simulink model "pam4"  (R2024a)
settings: Solver=VariableStepAuto  StartTime=0.0  StopTime=1  RelTol=1e-3
values from neighbouring files (symbols this model uses):
  channelCoeffs = [0.7,-0.2,0.1,0.3,0.2,-0.1]    [init.m]
  delay = span/2*M    (= 2)    [init.m]
  h = h/max(h)    [init.m]
  Rb = Rs*M    (= 7680000000)    [init.m]
  sps = 4    [init.m]
libraries: commdigbbndam3 x2, commchan3 x1, commrandsrc3 x1, commsink2 x1, dspadpt3 x1, dspsigops x1
settings Model: Creator=abc  LastModifiedBy=abc

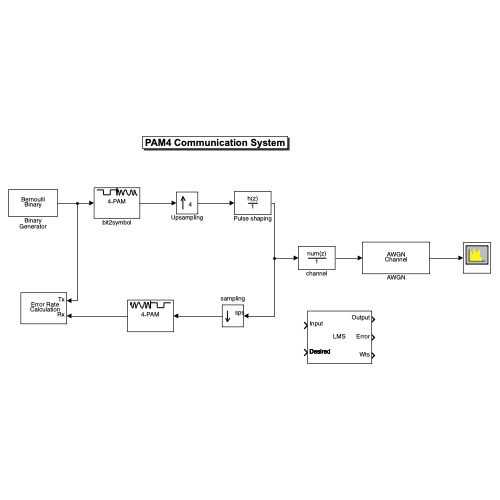
[thumbnail: Simulink's stored preview of the top-level diagram]
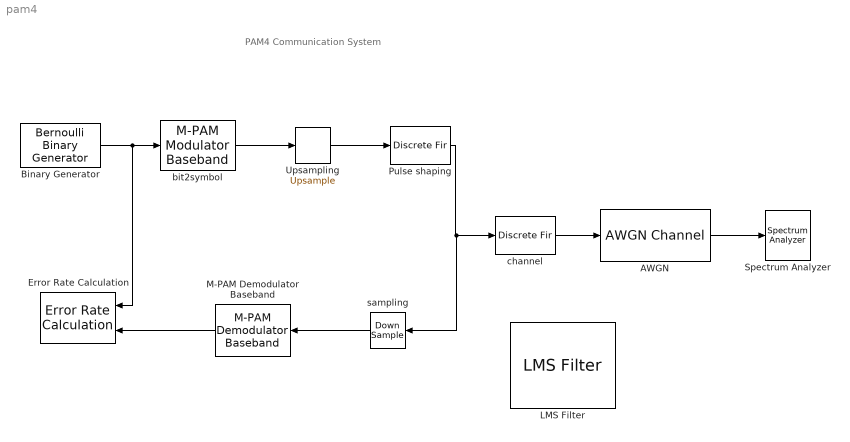
== system pam4 ==
  note: PAM4 Communication System
  AWGN : commchan3/AWGN Channel  LegacyMode=off  NoiseMethod="Signal to noise ratio  (Eb/No)"  noiseMode="Signal to noise ratio  (SNR)"  EbNo=EbN0  EsNo=10  SNR=10  BitsPerSymbol=M  SignalPower=signalPower  SamplesPerSymbol=sps  SymbolPeriod=1  VarianceSource=Parameter  Variance=1  RandomStream=Global stream  Seed=67  SimulateUsing=Interpreted execution
  Binary Generator : commrandsrc3/Bernoulli Binary Generator  ProbabilityOfZero=0.5  SeedSource=Auto  Seed=0  SampleTime=1/Rb  SamplesPerFrame=batchSize  OutputDataType=boolean  SimulateUsing=Interpreted execution
  Error Rate Calculation : commsink2/Error Rate Calculation  N=delay  st_delay=0  cp_mode=Entire frame  subframe=[]  PMode=Workspace  WsName=ErrorVec  RsMode2=off  stop=off  numErr=100  maxBits=1e6
  LMS Filter : dspadpt3/LMS Filter  Algo=LMS  L=16  stepflag=Dialog  mu=0.01  leakage=1.0  ic=0  Adapt=off  resetflag=None  weights=on  addnparflag=off  roundingMode=Floor  overflowMode=off
  M-PAM Demodulator Baseband : commdigbbndam3/M-PAM Demodulator Baseband  M=4  OutType=Bit  Dec=Gray  PowType=Min. distance between symbols  MinDist=2  AvgPow=1  PeakPow=1  outDtype1=boolean  outDtype2=Inherit via internal rule  denormFactorWordLen=16  denormFactorDataTypeStr=Inherit: Same word length as input  denormFactorLastDataTypeStr=Inherit: Same word length as input  prodOutWordLen=16  prodOutRoundingMode=Floor  prodOutOverflowMode=Wrap  prodOutOvFlMode=off  prodOutOvFlModeLastStrValue=off  sumWordLen=16
  Pulse shaping : DiscreteFir  Coefficients=h  InputProcessing=Columns as channels (frame based)
  Spectrum Analyzer : SpectrumAnalyzer  WindowPosition=[454.000000,177.000000,800.000000,500.000000,]  ScopeFrameLocation=window  Span=61440000000  StartFrequency=-30720000000  StopFrequency=30720000000  YLimits=[-73.48980676,24.64167876]
  Upsampling : dspsigops/Upsample  FactorSource=Dialog parameter  N=sps  Nmax=16  phase=0  InputProcessing=Columns as channels (frame based)  RateOptions=Enforce single-rate processing  ic=0  mode=Unused parameter value
  bit2symbol : commdigbbndam3/M-PAM Modulator Baseband  M=4  InType=Bit  Enc=Gray  PowType=Min. distance between symbols  MinDist=2  AvgPow=1  PeakPow=1  outDtype=double  outWordLen=16  outUDDataType=sfix(16)  outFracLenMode=Best precision  outFracLen=15  outDataTypeStr=double  outLastDataTypeStr=double
  channel : DiscreteFir  Coefficients=channelCoeffs  InputProcessing=Columns as channels (frame based)
  sampling : DownSample  N=sps
  wires:
  Binary Generator/1 -> Error Rate Calculation/1, bit2symbol/1
  bit2symbol/1 -> Upsampling/1
  Upsampling/1 -> Pulse shaping/1
  channel/1 -> AWGN/1
  AWGN/1 -> Spectrum Analyzer/1
  sampling/1 -> M-PAM Demodulator Baseband/1
  Pulse shaping/1 -> sampling/1, channel/1
  M-PAM Demodulator Baseband/1 -> Error Rate Calculation/2
